simulink model "bounding_spine_Simscape"  (R2024a)
settings: Solver=VariableStepAuto  StartTime=0.0  StopTime=30  RelTol=1e-2  AbsTol=1e-2
InitFcn:
  | run('initBusObjects.m');
  | run("parameters.m");
libraries: SignalEditorBlockLib x1
settings Model: Creator=Mechatronics  LastModifiedBy=heath
settings SolverCC: AutoInsertRateTranBlk=on

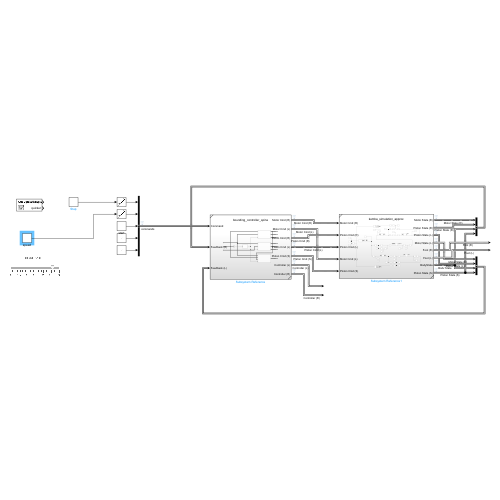
[thumbnail: Simulink's stored preview of the top-level diagram]
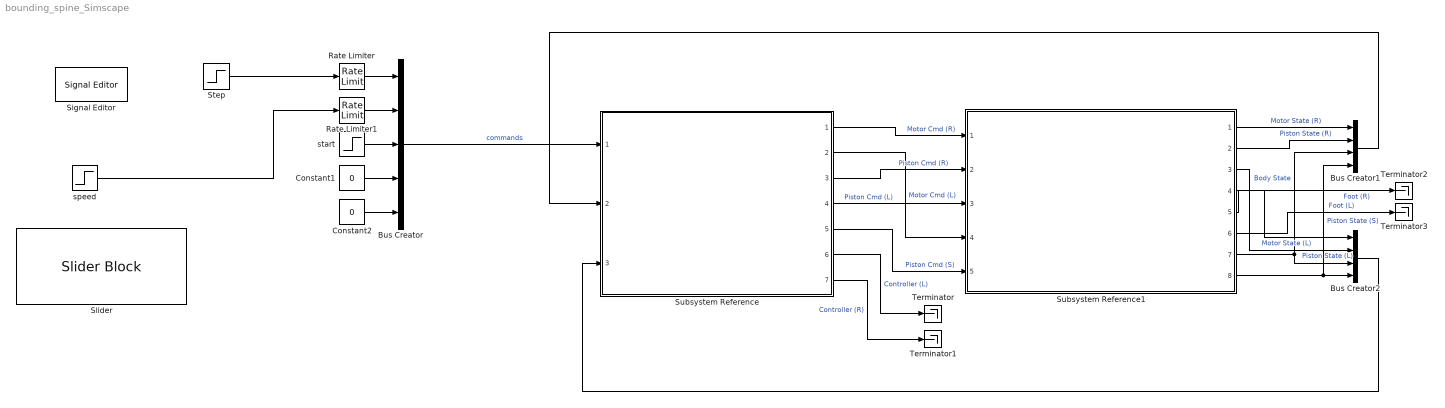
== system bounding_spine_Simscape ==
  Bus Creator : BusCreator  Inputs=5  OutDataTypeStr=Bus: Command
      settings: InheritFromInputs=off
  Bus Creator1 : BusCreator  Inputs=4  OutDataTypeStr=Bus: State
      settings: InheritFromInputs=off
  Bus Creator2 : BusCreator  Inputs=4  OutDataTypeStr=Bus: State
      settings: InheritFromInputs=off
  Constant1 : Constant  Value=0
  Constant2 : Constant  Value=0
  Rate Limiter : RateLimiter  RisingSlewLimit=0.05  FallingSlewLimit=-0.05  SampleTimeMode=inherited
  Rate Limiter1 : RateLimiter  RisingSlewLimit=0.18  FallingSlewLimit=-0.18  SampleTimeMode=inherited
  Signal Editor : SignalEditorBlockLib/Signal Editor  FileName=SpeedSteps.mat  ActiveScenario=UnactuatedSpine  ActiveSignal=point2steps  IsBus=off  OutputBusObjectStr=Bus: BusObject  SampleTime=0  Interpolate=off  ZeroCross=off  OutputAfterFinalValue=Setting to zero  Unit=inherit  PreserveSignalName=on  ApplySigPropsToAllScenarios=on  ApplySigPropsToAllSignals=off
  Slider : SliderBlock  ScaleMax=3
  Step : Step  Before=0.3  After=0.3  SampleTime=0
  Subsystem Reference : Subsystem  ReferencedSubsystem=bounding_controller_spine
  Subsystem Reference1 : Subsystem  ReferencedSubsystem=kemba_simulation_approx
  Terminator{,1..3} (4 alike) : Terminator
  speed : Step  Time=4  After=2.6  SampleTime=0
  start : Step  SampleTime=0
  wires:
  Subsystem Reference/1 -> Subsystem Reference1/1  "Motor Cmd (R)"
  Subsystem Reference/2 -> Subsystem Reference1/4  "Motor Cmd (L)"
  Subsystem Reference/3 -> Subsystem Reference1/2  "Piston Cmd (R)"
  Subsystem Reference/4 -> Subsystem Reference1/3  "Piston Cmd (L)"
  Subsystem Reference/5 -> Subsystem Reference1/5  "Piston Cmd (S)"
  Subsystem Reference/6 -> Terminator/1  "Controller (L)"
  Subsystem Reference/7 -> Terminator1/1  "Controller (R)"
  Subsystem Reference1/1 -> Bus Creator1/1  "Motor State (R)"
  Subsystem Reference1/2 -> Bus Creator1/2  "Piston State (R)"
  Subsystem Reference1/7 -> Bus Creator1/3, Bus Creator2/3  "Body State"
  Subsystem Reference1/8 -> Bus Creator2/4, Bus Creator1/4  "Piston State (S)"
  Bus Creator1/1 -> Subsystem Reference/2
  Subsystem Reference1/4 -> Bus Creator2/1  "Motor State (L)"
  Subsystem Reference1/3 -> Bus Creator2/2  "Piston State (L)"
  Bus Creator2/1 -> Subsystem Reference/3
  Subsystem Reference1/5 -> Terminator2/1  "Foot (R)"
  Subsystem Reference1/6 -> Terminator3/1  "Foot (L)"
  speed/1 -> Rate Limiter1/1
  Constant2/1 -> Bus Creator/5
  Rate Limiter/1 -> Bus Creator/1
  start/1 -> Bus Creator/3
  Constant1/1 -> Bus Creator/4
  Rate Limiter1/1 -> Bus Creator/2
  Step/1 -> Rate Limiter/1
  Bus Creator/1 -> Subsystem Reference/1  "commands"
